simulink model "leditbeat"  (Simulink 7.7)
settings: Solver=ode45  StartTime=0.0  StopTime=50.0  RelTol=1e-3
undefined symbols (not defined in the file or in its folder): dfilt, fdesignblkfcn, gcbh
libraries: simulink_extras x6, dspsigattribs x3, dspbuff3 x3, dspsrcs4 x2, dsparch4 x2, dspsnks4 x1
settings Model: Creator=Jx  LastModifiedBy=Jx

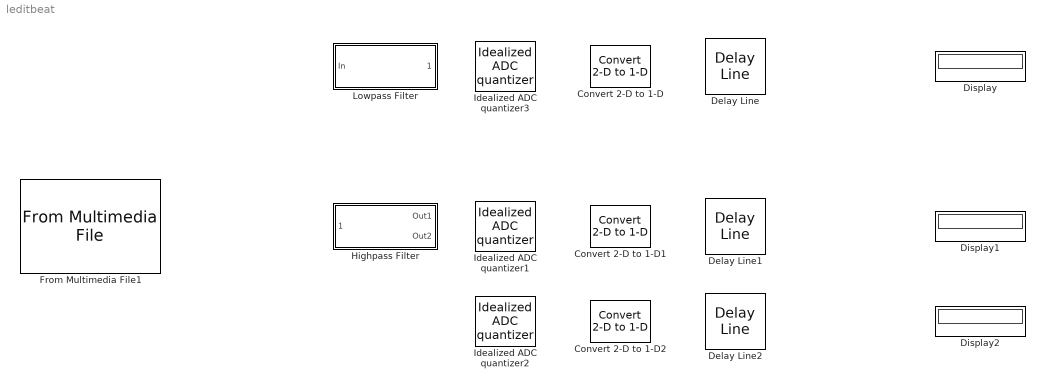
== system leditbeat ==
  Convert 2-D to 1-D : dspsigattribs/Convert 2-D to 1-D  SystemSampleTime=-1
  Convert 2-D to 1-D1 : dspsigattribs/Convert 2-D to 1-D  SystemSampleTime=-1
  Convert 2-D to 1-D2 : dspsigattribs/Convert 2-D to 1-D  SystemSampleTime=-1
  Delay Line : dspbuff3/Delay Line  siz=64  ic=0  directfeed=off  enable_output=off  hold_output=off  TreatMby1Signals=One channel
  Delay Line1 : dspbuff3/Delay Line  siz=64  ic=0  directfeed=off  enable_output=off  hold_output=off  TreatMby1Signals=One channel
  Delay Line2 : dspbuff3/Delay Line  siz=64  ic=0  directfeed=off  enable_output=off  hold_output=off  TreatMby1Signals=One channel
  Display : Display
  Display1 : Display
  Display2 : Display
  From Multimedia File1 : dspsrcs4/From Multimedia File  inputFilename=C:\Users\Jx\Desktop\jx\Music\01 Good Time.mp3  loop=on  numPlays=inf  outputStreams=Audio only  videoDataType=single  audioDataType=single  inheritSampleTime=on  userDefinedSampleTime=1/30  noAudioOutput=off  isIntensityVideo=off  fourcc=RGB  colorVideoFormat=Separate color signals  outputEOF=off  dataOrg=Column-major  audioFrameSize=1024  computeAudioFrameSize=off
  Highpass Filter : Subsystem  DialogController=fdesignblkfcn  DialogControllerArgs=DataTag4  InitFcn=fdesignblkfcn(gcbh, {'InitFcn'});
      settings: CopyFcn=fdesignblkfcn(gcbh, {'CopyFcn'});
      mask Type: Highpass Filter
      mask Description: Design a highpass filter
      mask Help: helpview(mapfilelocation('dsp'), 'dsphighpassfilter');
      mask Display: disp('Highpass')
  Idealized ADC quantizer1 : simulink_extras/Additional Discrete/Idealized ADC quantizer  SystemSampleTime=-1  NumberOfConverterBits=16  Vmin=0  Vmax=5  OutputDataType=int16  OutputNegativeValues=off
  Idealized ADC quantizer2 : simulink_extras/Additional Discrete/Idealized ADC quantizer  SystemSampleTime=-1  NumberOfConverterBits=16  Vmin=0  Vmax=5  OutputDataType=int16  OutputNegativeValues=off
  Idealized ADC quantizer3 : simulink_extras/Additional Discrete/Idealized ADC quantizer  SystemSampleTime=-1  NumberOfConverterBits=16  Vmin=0  Vmax=5  OutputDataType=int16  OutputNegativeValues=off
  Lowpass Filter : Subsystem  DialogController=fdesignblkfcn  DialogControllerArgs=DataTag12  InitFcn=fdesignblkfcn(gcbh, {'InitFcn'});
      settings: CopyFcn=fdesignblkfcn(gcbh, {'CopyFcn'});
      mask Type: Lowpass Filter
      mask Description: Design a lowpass filter
      mask Help: helpview(mapfilelocation('dsp'), 'dsplowpassfilter');
      mask Display: disp('Lowpass')

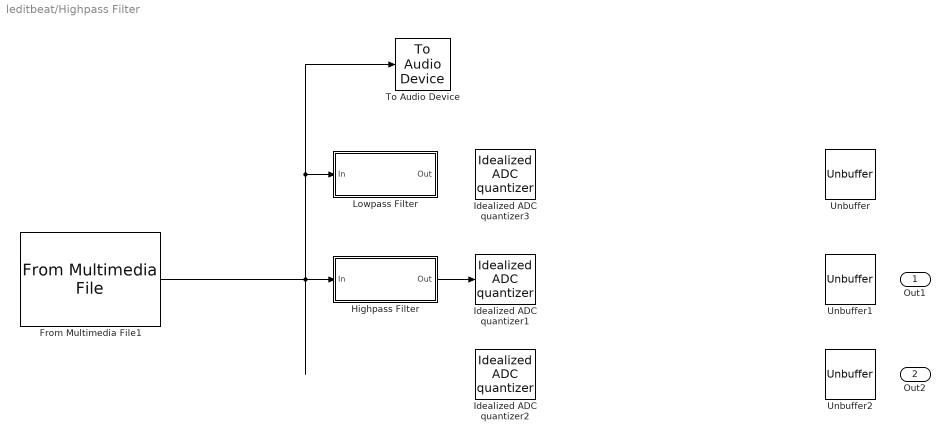
== system leditbeat/Highpass Filter ==
  From Multimedia File1 : dspsrcs4/From Multimedia File  inputFilename=C:\Users\Jx\Desktop\jx\Music\01 Good Time.mp3  loop=on  numPlays=inf  outputStreams=Audio only  videoDataType=single  audioDataType=single  inheritSampleTime=on  userDefinedSampleTime=1/30  noAudioOutput=off  isIntensityVideo=off  fourcc=RGB  colorVideoFormat=Separate color signals  outputEOF=off  dataOrg=Column-major  audioFrameSize=1024  computeAudioFrameSize=off
  Highpass Filter : Subsystem  DialogController=fdesignblkfcn  DialogControllerArgs=DataTag6  InitFcn=fdesignblkfcn(gcbh, {'InitFcn'});
      settings: CopyFcn=fdesignblkfcn(gcbh, {'CopyFcn'});
      mask Type: Highpass Filter
      mask Description: Design a highpass filter
      mask Help: helpview(mapfilelocation('dsp'), 'dsphighpassfilter');
      mask Display: disp('Highpass')
  Idealized ADC quantizer1 : simulink_extras/Additional Discrete/Idealized ADC quantizer  SystemSampleTime=-1  NumberOfConverterBits=8  Vmin=0  Vmax=255  OutputDataType=uint8  OutputNegativeValues=off
  Idealized ADC quantizer2 : simulink_extras/Additional Discrete/Idealized ADC quantizer  SystemSampleTime=-1  NumberOfConverterBits=8  Vmin=0  Vmax=255  OutputDataType=uint8  OutputNegativeValues=off
  Idealized ADC quantizer3 : simulink_extras/Additional Discrete/Idealized ADC quantizer  SystemSampleTime=-1  NumberOfConverterBits=16  Vmin=0  Vmax=5  OutputDataType=single  OutputNegativeValues=off
  Lowpass Filter : Subsystem  DialogController=fdesignblkfcn  DialogControllerArgs=DataTag9  InitFcn=fdesignblkfcn(gcbh, {'InitFcn'});
      settings: CopyFcn=fdesignblkfcn(gcbh, {'CopyFcn'});
      mask Type: Lowpass Filter
      mask Description: Design a lowpass filter
      mask Help: helpview(mapfilelocation('dsp'), 'dsplowpassfilter');
      mask Display: disp('Lowpass')
  To Audio Device : dspsnks4/To Audio Device  deviceName=Default  inheritSampleRate=on  sampleRate=44100  deviceDatatype=Determine from input data type  autoBufferSize=on  bufferSize=4096  queueDuration=1.0
  Unbuffer : Unbuffer  SampleBasedProcessing=Same as frame based
  Unbuffer1 : Unbuffer  SampleBasedProcessing=Same as frame based
  Unbuffer2 : Unbuffer  SampleBasedProcessing=Same as frame based
  Out1 : Outport
  Out2 : Outport  Port=2
  wires:
  From Multimedia File1/1 -> Highpass Filter/1(In), Lowpass Filter/1(In), To Audio Device/1
  Highpass Filter/1(Out) -> Idealized ADC quantizer1/1
  ? -> Idealized ADC quantizer2/1

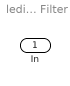
== system leditbeat/Lowpass Filter ==
  In : Inport

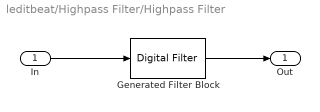
== system leditbeat/Highpass Filter/Highpass Filter ==
  In : Inport
  Generated Filter Block : dsparch4/Digital Filter  Tag=BlockMethodSubSystem  TypePopup=FIR (all zeros)  IIRFiltStruct=Direct form II transposed  AllPoleFiltStruct=Direct form  FIRFiltStruct=Direct form  CoeffSource=Specify via dialog  NumCoeffs=[-0.00171368266511037 0.00831437844808067 -0.0127173552334869 0.00556095179025034 0.00733971024255366 -0.00653104905017925 -0.0076900499697795 0.0090269831680985 0.00883886189950912 -0.0129607413537662 -0.0100749586672528 0.0185201740100089 0.011233354613589 -0.0263752483836136 -0.0122707821857659 0.0381809766923897 0.0131304259182936 -0.0582933593251923 -0.0137682959486481 0.102813257992074 0.0141678767738541 -0.317202552416035 0.485698046170518 -0.317202552416035 0.0141678767738541 0.102813257992074 -0.0137682959486481 -0.0582933593251923 0.0131304259182936 0.0381809766923897 -0.0122707821857659 -0.0263752483836136 0.011233354613589 0.0185201740100089 -0.0100749586672528 -0.0129607413537662 0.00883886189950912 0.0090269831680985 -0.0076900499697795 -0.00653104905017925 0.00733971024255366 0.00556095179025034 -0.0127173552334869 0.00831437844808067 -0.00171368266511037]  DenCoeffs=[1 0.1]  BiQuadCoeffs=[1 0.3 0.4 1 0.1 0.2]  LatticeCoeffs=[0.2 0.4]  denIgnore=on  FiltPerSampPopup=One filter per frame  IC=0  ICnum=0  ICden=0  roundingMode=Floor  overflowMode=off  ScaleValues=1  scaleValueFracLength=14  stageInFracLength=15  stageOutFracLength=15  FilterSource=Specify via dialog  dfiltObjectName=dfilt.dffir([1 2 1])  InputProcessing=Columns as channels (frame based)
  Out : Outport
  wires:
  Generated Filter Block/1 -> Out/1
  In/1 -> Generated Filter Block/1

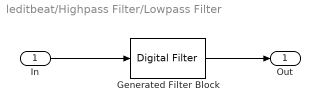
== system leditbeat/Highpass Filter/Lowpass Filter ==
  In : Inport
  Generated Filter Block : dsparch4/Digital Filter  Tag=BlockMethodSubSystem  TypePopup=FIR (all zeros)  IIRFiltStruct=Direct form II transposed  AllPoleFiltStruct=Direct form  FIRFiltStruct=Direct form  CoeffSource=Specify via dialog  NumCoeffs=[-0.00242287385232699 -0.00208324498207929 0.00677034464011864 0.016731945423489 0.0111170760810776 -0.00623114541414452 -0.00840161718602686 0.00925679761513803 0.0129828838088558 -0.010121234703279 -0.0182735187337825 0.011431962071778 0.0261758885804076 -0.012489027835323 -0.0379966231454636 0.0133889451993669 0.0581554658147299 -0.0140480435158089 -0.102724668578822 0.0144622757712384 0.317166497217695 0.485387646787325 0.317166497217695 0.0144622757712384 -0.102724668578822 -0.0140480435158089 0.0581554658147299 0.0133889451993669 -0.0379966231454636 -0.012489027835323 0.0261758885804076 0.011431962071778 -0.0182735187337825 -0.010121234703279 0.0129828838088558 0.00925679761513803 -0.00840161718602686 -0.00623114541414452 0.0111170760810776 0.016731945423489 0.00677034464011864 -0.00208324498207929 -0.00242287385232699]  DenCoeffs=[1 0.1]  BiQuadCoeffs=[1 0.3 0.4 1 0.1 0.2]  LatticeCoeffs=[0.2 0.4]  denIgnore=on  FiltPerSampPopup=One filter per frame  IC=0  ICnum=0  ICden=0  roundingMode=Floor  overflowMode=off  ScaleValues=1  scaleValueFracLength=14  stageInFracLength=15  stageOutFracLength=15  FilterSource=Specify via dialog  dfiltObjectName=dfilt.dffir([1 2 1])  InputProcessing=Columns as channels (frame based)
  Out : Outport
  wires:
  In/1 -> Generated Filter Block/1
  Generated Filter Block/1 -> Out/1
